simulink model "LPF"  (R2023b)
settings: Solver=FixedStepAuto  StartTime=0.0  StopTime=100  FixedStep=Tsim  RelTol=1e-3
InitFcn:
  | Tsim = 10e-6;   % Simulation Step time
  | 
  | % Ts is the sample time of discrete LPF
  | % 10e-6 for inuput_signal = 4
  | Ts = 0.1; %10e-6; %2.1;
  | 
  | % LPF Time Constant
  | Tau = 1;
  | 
  | % 1: constant 1; 2: step changes;
  | % 3: Ramp; 4:Sinusoidal; 5: pulse
  | input_signal = 2;
  | 
  | % 0 for all input_signals except 4
  | freq = 0;
  | % Frequency modulation index fsw/f
  | mf = 60000;
  | Gain = sqrt(1+(2*pi*freq)^2);
  | 
  | alpha = 1-exp(-Ts/Tau);
libraries: simulink x1
settings Model: Creator=Administrator  LastModifiedBy=Administrator

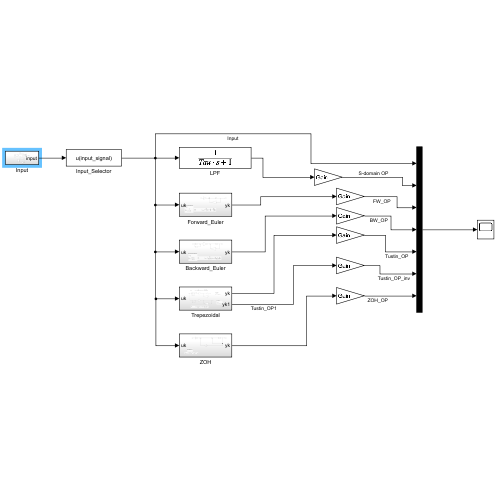
[thumbnail: Simulink's stored preview of the top-level diagram]
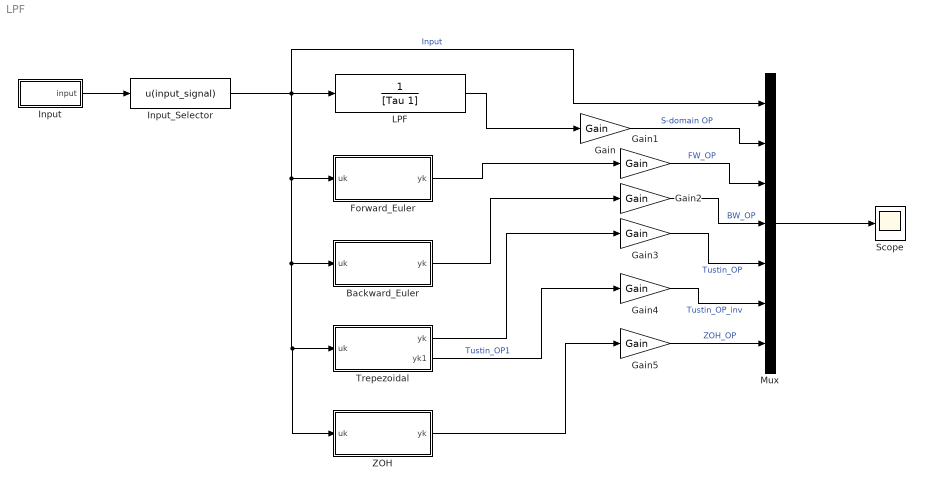
== system LPF ==
  Backward_Euler : Subsystem
  Forward_Euler : Subsystem
  Gain{,1..5} (6 alike) : Gain  Gain=Gain
  Input : Subsystem
  Input_Selector : Fcn  Expr=u(input_signal)
  LPF : TransferFcn  Denominator=[Tau 1]
  Mux : Mux  Inputs=7
  Scope : Scope
  Trepezoidal : Subsystem
  ZOH : Subsystem
  wires:
  Mux/1 -> Scope/1
  Input_Selector/1 -> Mux/1, ZOH/1(uk), Trepezoidal/1(uk), Backward_Euler/1(uk), Forward_Euler/1(uk), LPF/1  "Input"
  LPF/1 -> Gain/1
  Forward_Euler/1(yk) -> Gain1/1
  Backward_Euler/1(yk) -> Gain2/1
  Trepezoidal/1(yk) -> Gain3/1
  Trepezoidal/2(yk1) -> Gain4/1  "Tustin_OP1"
  Gain/1 -> Mux/2  "S-domain OP"
  Gain1/1 -> Mux/3  "FW_OP"
  Gain2/1 -> Mux/4  "BW_OP"
  Gain3/1 -> Mux/5  "Tustin_OP"
  Gain4/1 -> Mux/6  "Tustin_OP_inv"
  Input/1(input) -> Input_Selector/1
  ZOH/1(yk) -> Gain5/1
  Gain5/1 -> Mux/7  "ZOH_OP"

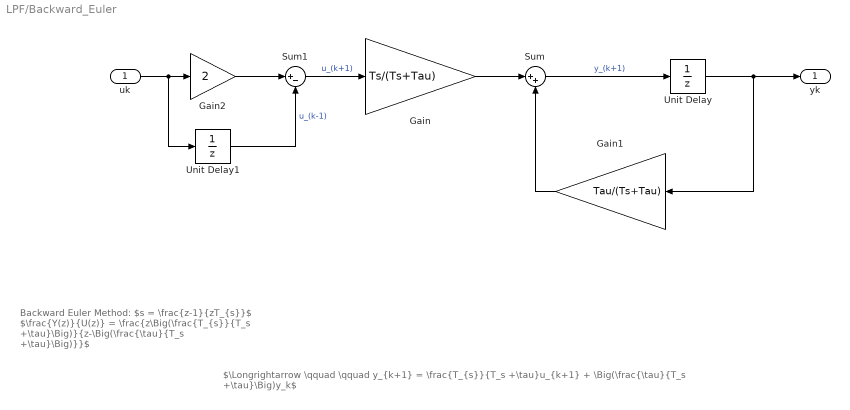
== system LPF/Backward_Euler ==
  note: Backward Euler Method:
      | $s = \frac{z-1}{zT_{s}}$
      | $\frac{Y(z)}{U(z)} = \frac{z\Big(\frac{T_{s}}{T_s +\tau}\Big)}{z-\Big(\frac{\tau}{T_s +\tau}\Big)}}$
  note: $\Longrightarrow \qquad \qquad y_{k+1} = \frac{T_{s}}{T_s +\tau}u_{k+1} + \Big(\frac{\tau}{T_s +\tau}\Big)y_k$
  uk : Inport
  Gain : Gain  Gain=Ts/(Ts+Tau)
  Gain1 : Gain  Gain=Tau/(Ts+Tau)
  Gain2 : Gain  Gain=2
  Sum : Sum  Inputs=|++
  Sum1 : Sum  Inputs=|+-
  Unit Delay : UnitDelay  SampleTime=Ts  HasFrameUpgradeWarning=on
  Unit Delay1 : UnitDelay  SampleTime=Ts  HasFrameUpgradeWarning=on
  yk : Outport
  wires:
  Unit Delay/1 -> Gain1/1, yk/1
  Sum/1 -> Unit Delay/1  "y_(k+1)"
  Gain1/1 -> Sum/2
  Gain/1 -> Sum/1
  uk/1 -> Unit Delay1/1, Gain2/1
  Gain2/1 -> Sum1/1
  Unit Delay1/1 -> Sum1/2  "u_(k-1)"
  Sum1/1 -> Gain/1  "u_(k+1)"

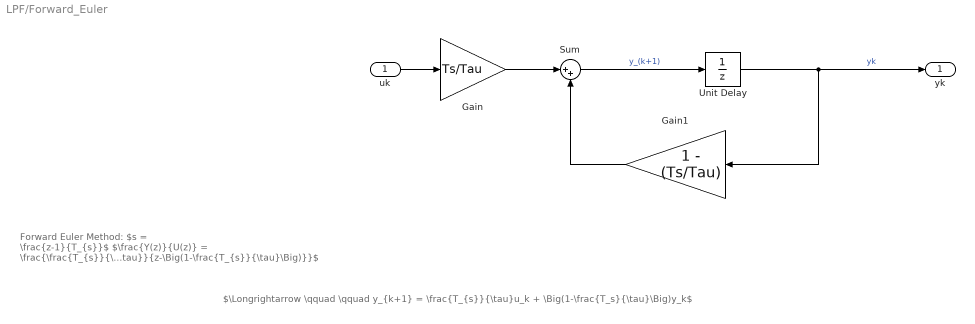
== system LPF/Forward_Euler ==
  note: $\Longrightarrow \qquad \qquad y_{k+1} = \frac{T_{s}}{\tau}u_k + \Big(1-\frac{T_s}{\tau}\Big)y_k$
  note: Forward Euler Method:
      | $s = \frac{z-1}{T_{s}}$
      | $\frac{Y(z)}{U(z)} = \frac{\frac{T_{s}}{\tau}}{z-\Big(1-\frac{T_{s}}{\tau}\Big)}}$
  uk : Inport
  Gain : Gain  Gain=Ts/Tau
  Gain1 : Gain  Gain=1 - (Ts/Tau)
  Sum : Sum  Inputs=|++
  Unit Delay : UnitDelay  SampleTime=Ts  HasFrameUpgradeWarning=on
  yk : Outport
  wires:
  Gain/1 -> Sum/1
  Gain1/1 -> Sum/2
  Sum/1 -> Unit Delay/1  "y_(k+1)"
  uk/1 -> Gain/1
  Unit Delay/1 -> Gain1/1, yk/1  "yk"

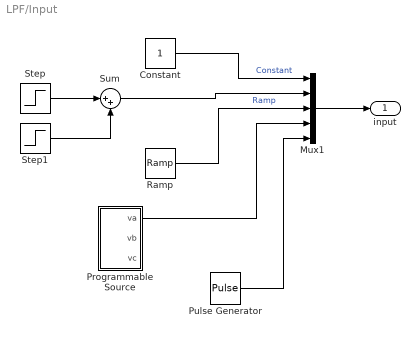
== system LPF/Input ==
  Constant : Constant
  Mux1 : Mux  Inputs=5
  Programmable Source : Subsystem  mask(DSOGI - PLL){f=freq, V=1/sqrt(2)}
      mask prompts: f "Fundamental grid frequency (f) in Hz"; V "Fundamental grid voltage (V) in RMS volts"
      mask help: Programmable source generates a signal with fundamental and odd harmonic signals upto 13th frequency component.
  Pulse Generator : DiscretePulseGenerator  PulseType=Time based  Period=10  PulseWidth=50
  Ramp : simulink/Sources/Ramp  slope=1  start=0  InitialOutput=0
  Step : Step  Time=0  SampleTime=0
  Step1 : Step  Time=20  SampleTime=0
  Sum : Sum  Inputs=|++
  input : Outport
  wires:
  Ramp/1 -> Mux1/3  "Ramp"
  Constant/1 -> Mux1/1  "Constant"
  Step1/1 -> Sum/2
  Mux1/1 -> input/1
  Programmable Source/1(va) -> Mux1/4
  Step/1 -> Sum/1
  Sum/1 -> Mux1/2
  Pulse Generator/1 -> Mux1/5

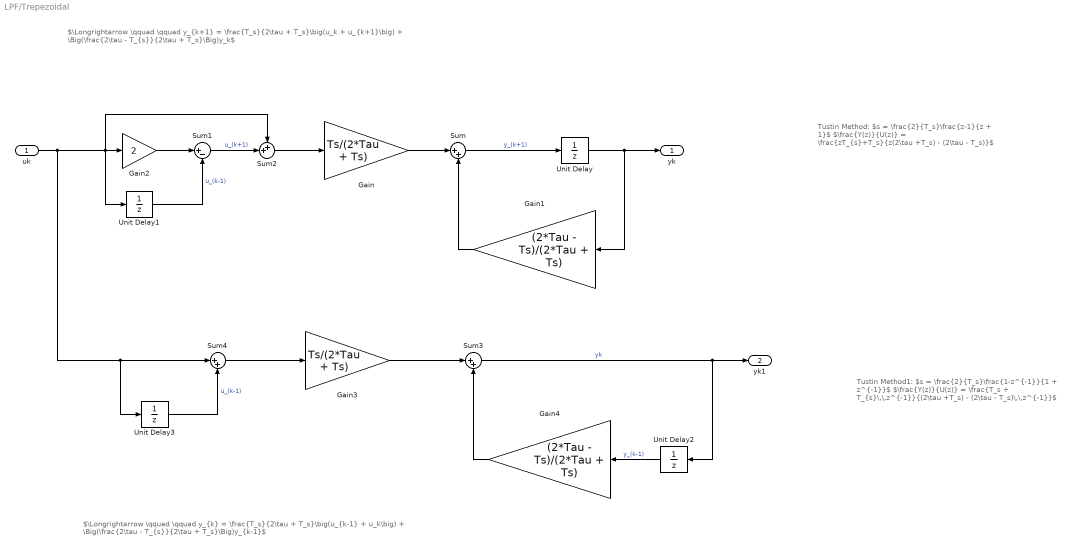
== system LPF/Trepezoidal ==
  note: $\Longrightarrow \qquad \qquad y_{k+1} = \frac{T_s}{2\tau + T_s}\big(u_k + u_{k+1}\big) + \Big(\frac{2\tau - T_{s}}{2\tau + T_s}\Big)y_k$
  note: Tustin Method:
      | $s = \frac{2}{T_s}\frac{z-1}{z + 1}$
      | $\frac{Y(z)}{U(z)} = \frac{zT_{s}+T_s}{z(2\tau +T_s) - (2\tau - T_s)}$
  note: Tustin Method1:
      | $s = \frac{2}{T_s}\frac{1-z^{-1}}{1 + z^{-1}}$
      | $\frac{Y(z)}{U(z)} = \frac{T_s + T_{s}\,\,z^{-1}}{(2\tau +T_s) - (2\tau - T_s)\,\,z^{-1}}$
  note: $\Longrightarrow \qquad \qquad y_{k} = \frac{T_s}{2\tau + T_s}\big(u_{k-1} + u_k\big) + \Big(\frac{2\tau - T_{s}}{2\tau + T_s}\Big)y_{k-1}$
  uk : Inport
  Gain : Gain  Gain=Ts/(2*Tau + Ts)
  Gain1 : Gain  Gain=(2*Tau - Ts)/(2*Tau + Ts)
  Gain2 : Gain  Gain=2
  Gain3 : Gain  Gain=Ts/(2*Tau + Ts)
  Gain4 : Gain  Gain=(2*Tau - Ts)/(2*Tau + Ts)
  Sum : Sum  Inputs=|++
  Sum1 : Sum  Inputs=|+-
  Sum2 : Sum  Inputs=++|
  Sum3 : Sum  Inputs=|++
  Sum4 : Sum  Inputs=|++
  Unit Delay{,1..3} (4 alike) : UnitDelay  SampleTime=Ts  HasFrameUpgradeWarning=on
  yk : Outport
  yk1 : Outport  Port=2
  wires:
  Unit Delay/1 -> Gain1/1, yk/1
  Sum/1 -> Unit Delay/1  "y_(k+1)"
  Gain1/1 -> Sum/2
  Gain/1 -> Sum/1
  Gain2/1 -> Sum1/1
  Unit Delay1/1 -> Sum1/2  "u_(k-1)"
  Sum1/1 -> Sum2/2  "u_(k+1)"
  Sum2/1 -> Gain/1
  Unit Delay3/1 -> Sum4/2  "u_(k-1)"
  uk/1 -> Sum4/1, Unit Delay3/1, Sum2/1, Unit Delay1/1, Gain2/1
  Sum3/1 -> Unit Delay2/1, yk1/1  "yk"
  Gain4/1 -> Sum3/2
  Gain3/1 -> Sum3/1
  Sum4/1 -> Gain3/1
  Unit Delay2/1 -> Gain4/1  "y_(k-1)"

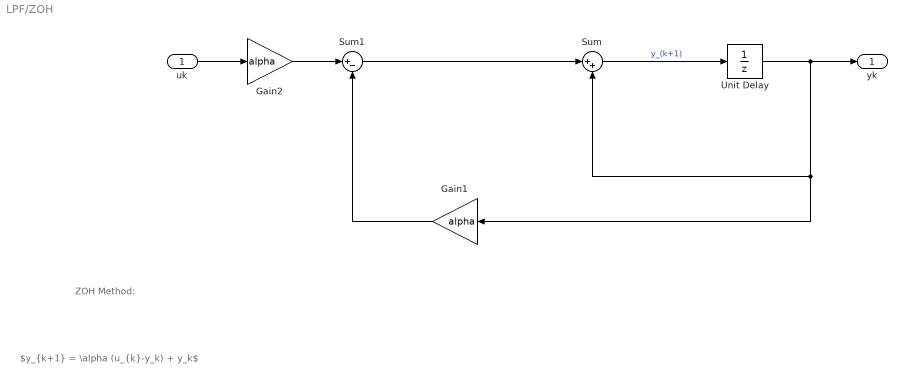
== system LPF/ZOH ==
  note: ZOH Method:
  note: $y_{k+1} = \alpha (u_{k}-y_k) + y_k$
  uk : Inport
  Gain1 : Gain  Gain=alpha
  Gain2 : Gain  Gain=alpha
  Sum : Sum  Inputs=|++
  Sum1 : Sum  Inputs=|+-
  Unit Delay : UnitDelay  SampleTime=Ts  HasFrameUpgradeWarning=on
  yk : Outport
  wires:
  Sum/1 -> Unit Delay/1  "y_(k+1)"
  Unit Delay/1 -> Gain1/1, Sum/2, yk/1
  uk/1 -> Gain2/1
  Gain2/1 -> Sum1/1
  Gain1/1 -> Sum1/2
  Sum1/1 -> Sum/1

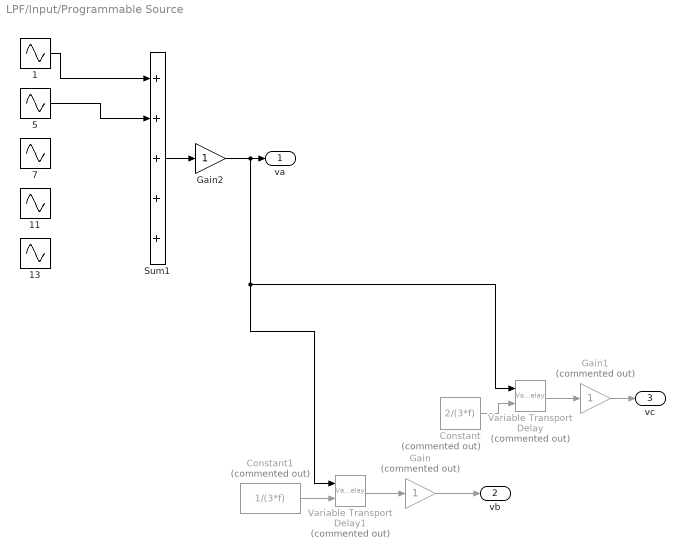
== system LPF/Input/Programmable Source ==
  1 : Sin  Amplitude=V*sqrt(2)  Frequency=2*pi*f  Phase=0*pi/2  SampleTime=0
  11 : Sin  Amplitude=V*sqrt(2)/11  Frequency=2*pi*11*f  Phase=0*pi/2  SampleTime=0
  13 : Sin  Amplitude=V*sqrt(2)/13  Frequency=2*pi*13*f  Phase=0*pi/2  SampleTime=0
  5 : Sin  Amplitude=V*sqrt(2)/5  Frequency=2*pi*mf*f  Phase=0*pi/2  SampleTime=0
  7 : Sin  Amplitude=V*sqrt(2)/7  Frequency=2*pi*7*f  Phase=0*pi/2  SampleTime=0
  Constant : Constant  Commented=on  Value=2/(3*f)
  Constant1 : Constant  Commented=on  Value=1/(3*f)
  Gain : Gain  Commented=on
  Gain1 : Gain  Commented=on
  Gain2 : Gain
  Sum1 : Sum  Inputs=+++++
  Variable Transport Delay : VariableTransportDelay  Commented=on  VariableDelayType=Variable transport delay  MaximumDelay=10
  Variable Transport Delay1 : VariableTransportDelay  Commented=on  VariableDelayType=Variable transport delay  MaximumDelay=10
  va : Outport  VectorParamsAs1DForOutWhenUnconnected=off
  vb : Outport  Port=2  VectorParamsAs1DForOutWhenUnconnected=off
  vc : Outport  Port=3  VectorParamsAs1DForOutWhenUnconnected=off
  wires:
  Constant1/1 -> Variable Transport Delay1/2
  Constant/1 -> Variable Transport Delay/2
  Variable Transport Delay1/1 -> Gain/1
  Variable Transport Delay/1 -> Gain1/1
  Gain/1 -> vb/1
  Gain1/1 -> vc/1
  1/1 -> Sum1/1
  Gain2/1 -> Variable Transport Delay1/1, Variable Transport Delay/1, va/1
  5/1 -> Sum1/2
  Sum1/1 -> Gain2/1
